simulink model "Understanding_Control_Systems_2"  (R2017b)
settings: Solver=VariableStepAuto  StartTime=0.0  StopTime=400  RelTol=1e-3
PreLoadFcn:
  | Car=Simulink.Variant('vehicleType==1')
  | SportsCar=Simulink.Variant('vehicleType==2')
  | Truck=Simulink.Variant('vehicleType==3')
  | 
  | vehicleType=1
libraries: MeldasLibrary x3
settings Model: Creator=mulusoy  LastModifiedBy=mulusoy
settings CodeAppCC: StateflowObjectComments=on
settings ConfigComp: CovMetricSettings=dswe

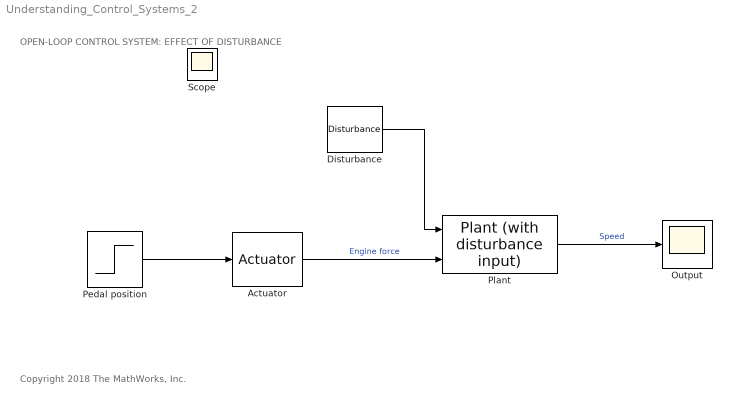
== system Understanding_Control_Systems_2 ==
  note: Copyright 2018 The MathWorks, Inc.
  note: OPEN-LOOP CONTROL SYSTEM: EFFECT OF DISTURBANCE
  Actuator : MeldasLibrary/Actuator  SystemSampleTime=-1
      settings: SourceProductName=Melda's Library
  Disturbance : MeldasLibrary/Disturbance  SystemSampleTime=-1
      settings: SourceProductName=Melda's Library
  Output : Scope
  Pedal position : Step  Time=5  After=pi/6  SampleTime=0
  Plant : MeldasLibrary/Plant (with disturbance input)  vehicleType=Car
      settings: SourceProductName=Melda's Library
  Scope : Scope
  wires:
  Pedal position/1 -> Actuator/1
  Actuator/1 -> Plant/2  "Engine force"
  Plant/1 -> Output/1  "Speed"
  Disturbance/1 -> Plant/1
